simulink model "vjezba5"  (Simulink 6.5)
settings: Solver=ode45  StartTime=0.0  StopTime=5.0  RelTol=1e-6
settings Model: Creator=im42741  LastModifiedBy=im42741

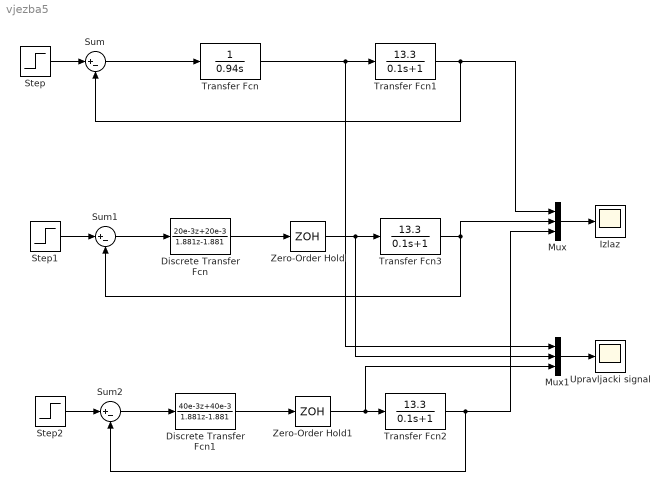
== system vjezba5 ==
  Discrete Transfer Fcn : DiscreteTransferFcn  Numerator=[20e-3 20e-3]  Denominator=[1.881 -1.881]  SampleTime=20e-3
  Discrete Transfer Fcn1 : DiscreteTransferFcn  Numerator=[40e-3 40e-3]  Denominator=[1.881 -1.881]  SampleTime=40e-3
  Izlaz : Scope
  Mux : Mux  Inputs=3
  Mux1 : Mux  Inputs=3
  Step : Step  Time=0  SampleTime=0
  Step1 : Step  Time=0  SampleTime=0
  Step2 : Step  Time=0  SampleTime=0
  Sum : Sum  Inputs=|+-
  Sum1 : Sum  Inputs=|+-
  Sum2 : Sum  Inputs=|+-
  Transfer Fcn : TransferFcn  Denominator=[0.94 0]
  Transfer Fcn1 : TransferFcn  Numerator=[13.3]  Denominator=[0.1 1]
  Transfer Fcn2 : TransferFcn  Numerator=[13.3]  Denominator=[0.1 1]
  Transfer Fcn3 : TransferFcn  Numerator=[13.3]  Denominator=[0.1 1]
  Upravljacki signal : Scope
      settings: SaveName=ScopeData2
  Zero-Order Hold : ZeroOrderHold  SampleTime=20e-3
  Zero-Order Hold1 : ZeroOrderHold  SampleTime=40e-3
  wires:
  Transfer Fcn/1 -> Transfer Fcn1/1, Mux1/1
  Sum/1 -> Transfer Fcn/1
  Transfer Fcn1/1 -> Sum/2, Mux/1
  Step/1 -> Sum/1
  Sum1/1 -> Discrete Transfer Fcn/1
  Transfer Fcn3/1 -> Sum1/2, Mux/2
  Step1/1 -> Sum1/1
  Zero-Order Hold/1 -> Transfer Fcn3/1, Mux1/2
  Discrete Transfer Fcn/1 -> Zero-Order Hold/1
  Sum2/1 -> Discrete Transfer Fcn1/1
  Transfer Fcn2/1 -> Sum2/2, Mux/3
  Step2/1 -> Sum2/1
  Zero-Order Hold1/1 -> Transfer Fcn2/1, Mux1/3
  Discrete Transfer Fcn1/1 -> Zero-Order Hold1/1
  Mux/1 -> Izlaz/1
  Mux1/1 -> Upravljacki signal/1
